simulink model "IEEE39BusSystem"  (R2025a)
settings: Solver=FixedStepDiscrete  StartTime=0.0  StopTime=15  FixedStep=Ts  MaxStep=1e-4  RelTol=1e-3
PreLoadFcn:
  | Ts = 1/60;
  | EnPSS = 1;
undefined symbols (not defined in the file or in its folder): Gen1, Gen10, Gen2, Gen3, Gen4, Gen5, Gen6, Gen7, Gen8, Gen9, Load12, Load15, Load16, Load18, Load20, Load21, Load23, Load24, Load25, Load26, Load27, Load28, Load29, Load3, Load31, Load39, Load4, Load7, Load8
libraries: ee_lib x197, fl_lib x97, nesl_utility x91, eeGeneralControl x20, eeSmAC1C x10, eeSmPSS1A x10
(part 1 of 6)
CloseFcn:
  | try,close(h1_IEEE39BusSystem),end
  | clear h1_IEEE39BusSystem
  | clear tout simlog_IEEE39BusSystem
Description:
  | IEEE 39-Bus System
settings Model: Creator=The MathWorks, Inc.  LastModifiedBy=The MathWorks, Inc.
settings SolverCC: MaxZcPerStep=1.0
settings DataIOCC: SaveFormat=Array  SaveOutput=off  DSMLogging=off  SaveTime=off  ReturnWorkspaceOutputs=off  SignalLoggingName=logsout_IEEE39BusSystem
settings OptimizationCC: ReuseModelBlockBuffer=off
settings ModelReferenceCC: EnableRefExpFcnMdlSchedulingChecks=on
settings RTWCC: GPUComputeCapability=3.5
settings SimscapeCC: SimscapeLogType=all  SimscapeLogSimulationStatistics=on  SimscapeLogName=simlog_IEEE39BusSystem  SimscapeLogDataHistory=10000.0

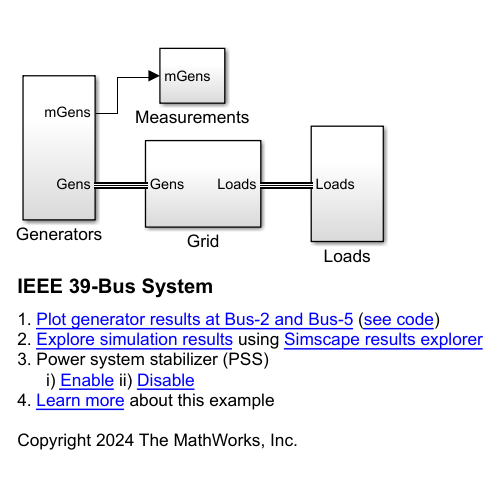
[thumbnail: Simulink's stored preview of the top-level diagram]
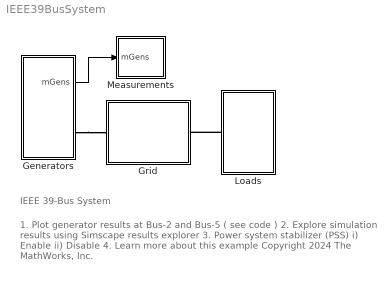
== system IEEE39BusSystem ==
  note: IEEE 39-Bus System
  note: 1. Plot generator results at Bus-2 and Bus-5 ( see code )
      | 2. Explore simulation results using Simscape results explorer
      | 3. Power system stabilizer (PSS)
      | i) Enable ii) Disable
      | 4. Learn more about this example
      |
      | Copyright 2024 The MathWorks, Inc.
  Generators : Subsystem
  Grid : Subsystem
  Loads : Subsystem
  Measurements : Subsystem
  wires:
  Generators/1(mGens) -> Measurements/1(mGens)
  connections:
  Generators/RConn1 -- Grid/LConn1
  Loads/LConn1 -- Grid/RConn1

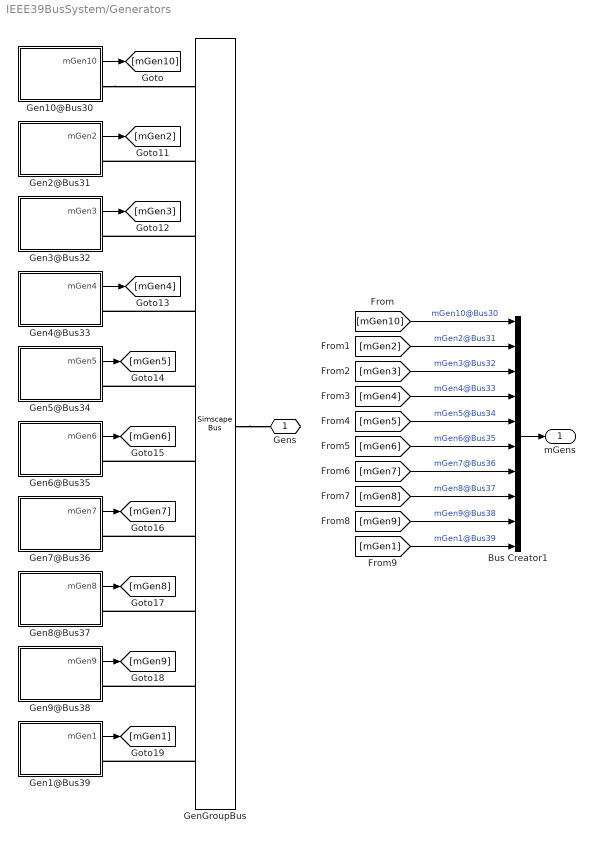
== system IEEE39BusSystem/Generators ==
  Bus Creator1 : BusCreator  Inputs=10
  Gen10@Bus30 : Subsystem
  Gen1@Bus39 : Subsystem
  Gen2@Bus31 : Subsystem
  Gen3@Bus32 : Subsystem
  Gen4@Bus33 : Subsystem
  Gen5@Bus34 : Subsystem
  Gen6@Bus35 : Subsystem
  Gen7@Bus36 : Subsystem
  Gen8@Bus37 : Subsystem
  Gen9@Bus38 : Subsystem
  GenGroupBus : SimscapeBus  HierarchyStrings=Gen10;Gen2;Gen3;Gen4;Gen5;Gen6;Gen7;Gen8;Gen9;Gen1
  Gens : PMIOPort  Side=Right
  mGens : Outport
  wires:
  Gen10@Bus30/1(mGen10) -> [mGen10]
  [mGen10] -> Bus Creator1/1  "mGen10@Bus30"
  [mGen2] -> Bus Creator1/2  "mGen2@Bus31"
  [mGen3] -> Bus Creator1/3  "mGen3@Bus32"
  [mGen4] -> Bus Creator1/4  "mGen4@Bus33"
  [mGen1] -> Bus Creator1/10  "mGen1@Bus39"
  [mGen9] -> Bus Creator1/9  "mGen9@Bus38"
  [mGen8] -> Bus Creator1/8  "mGen8@Bus37"
  [mGen7] -> Bus Creator1/7  "mGen7@Bus36"
  [mGen6] -> Bus Creator1/6  "mGen6@Bus35"
  [mGen5] -> Bus Creator1/5  "mGen5@Bus34"
  Bus Creator1/1 -> mGens/1
  Gen8@Bus37/1(mGen8) -> [mGen8]
  Gen5@Bus34/1(mGen5) -> [mGen5]
  Gen4@Bus33/1(mGen4) -> [mGen4]
  Gen1@Bus39/1(mGen1) -> [mGen1]
  Gen9@Bus38/1(mGen9) -> [mGen9]
  Gen7@Bus36/1(mGen7) -> [mGen7]
  Gen3@Bus32/1(mGen3) -> [mGen3]
  Gen6@Bus35/1(mGen6) -> [mGen6]
  Gen2@Bus31/1(mGen2) -> [mGen2]
  connections:
  Gen10@Bus30/RConn1 -- GenGroupBus/LConn1
  GenGroupBus/RConn1 -- Gens/RConn1
  GenGroupBus/LConn5 -- Gen5@Bus34/RConn1
  GenGroupBus/LConn8 -- Gen8@Bus37/RConn1
  GenGroupBus/LConn2 -- Gen2@Bus31/RConn1
  GenGroupBus/LConn7 -- Gen7@Bus36/RConn1
  GenGroupBus/LConn3 -- Gen3@Bus32/RConn1
  GenGroupBus/LConn10 -- Gen1@Bus39/RConn1
  GenGroupBus/LConn9 -- Gen9@Bus38/RConn1
  GenGroupBus/LConn4 -- Gen4@Bus33/RConn1
  GenGroupBus/LConn6 -- Gen6@Bus35/RConn1
